simulink library "MyLib"  (R2024a)
settings: Solver=VariableStepAuto  StartTime=0.0  StopTime=10.0  RelTol=1e-3
values from neighbouring files (symbols this model uses):
  cnt_min = 10    [TX_PM_MODEL_Setup.m]
  cnt_n_bits = 9    [TX_PM_MODEL_Setup.m]
  R = 0.2    [TX_PM_MODEL_Setup.m]
  tcmp = 5    [TX_PM_MODEL_Setup.m]
undefined symbols (not defined in the file or in its folder): VDD_DRIVE
libraries: fl_lib x12, nesl_utility x7, $bdroot x3, ee_lib x1, spsTriangleGeneratorLib x1
settings Model: Creator=ciano  LastModifiedBy=ciano

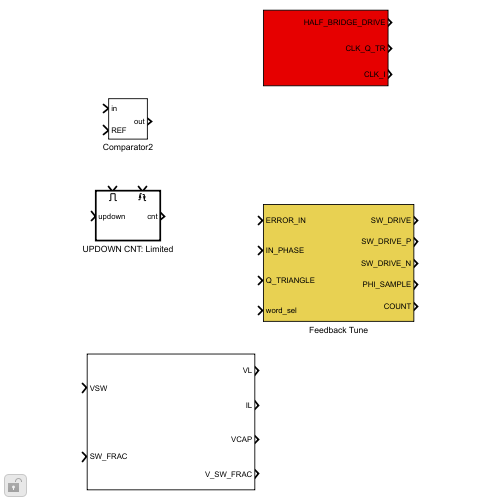
[thumbnail: Simulink's stored preview of the top-level diagram]
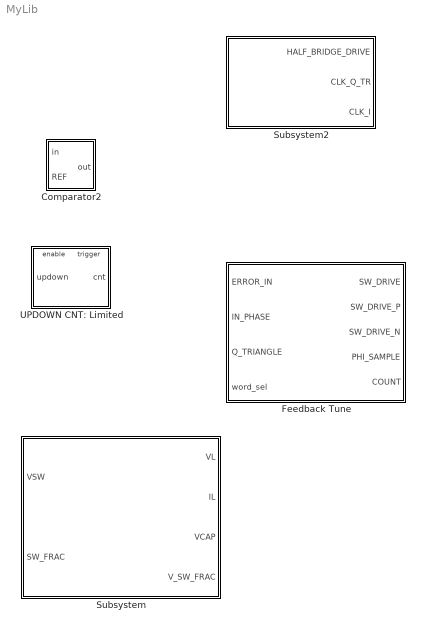
== system MyLib ==
  Comparator2 : Subsystem
  Feedback Tune : Subsystem
  Subsystem : Subsystem
  Subsystem2 : Subsystem
  UPDOWN CNT: Limited : Subsystem

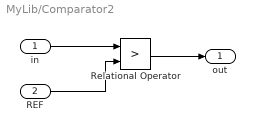
== system MyLib/Comparator2 ==
  in : Inport
  REF : Inport  Port=2
  Relational Operator : RelationalOperator  Operator=>  OutDataTypeStr=boolean  RndMeth=Simplest  InputSameDT=off
  out : Outport
  wires:
  in/1 -> Relational Operator/1
  Relational Operator/1 -> out/1
  REF/1 -> Relational Operator/2

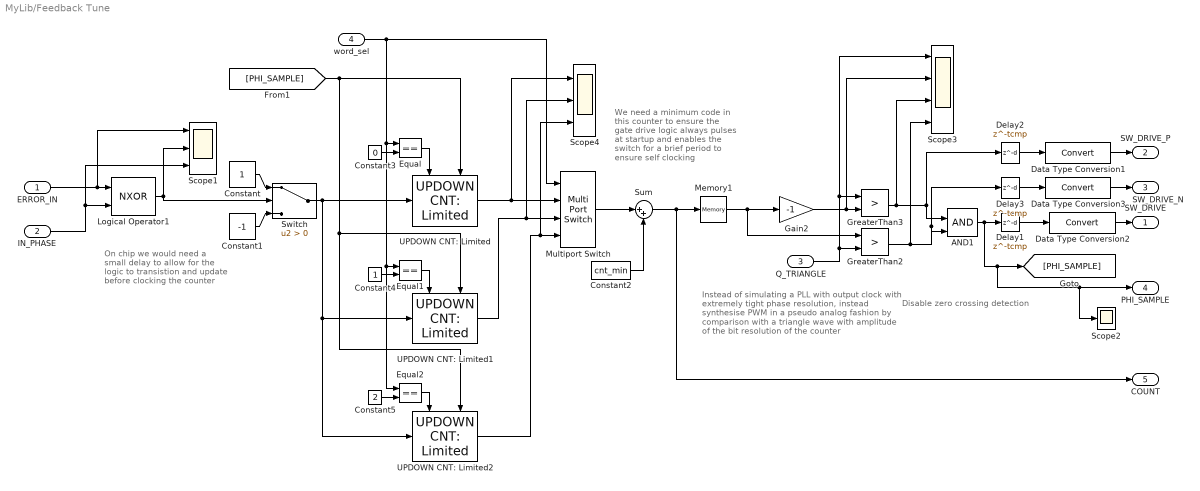
== system MyLib/Feedback Tune ==
  note: On chip we would need a small delay to allow for the logic to transistion and update before clocking the counter
  note: Instead of simulating a PLL with output clock with extremely tight phase resolution, instead synthesise PWM in a pseudo analog fashion by comparison with a triangle wave with amplitude of the bit resolution of the counter
  note: Disable zero crossing detection
  note: We need a minimum code in this counter to ensure the gate drive logic always pulses at startup and enables the switch for a brief period to ensure self clocking
  ERROR_IN : Inport
  IN_PHASE : Inport  Port=2
  Q_TRIANGLE : Inport  Port=3
  word_sel : Inport  Port=4
  AND1 : Logic  IconShape=distinctive  AllPortsSameDT=off  OutDataTypeStr=boolean
  Constant : Constant
  Constant1 : Constant  Value=-1
  Constant2 : Constant  Value=cnt_min
  Constant3 : Constant  Value=0
  Constant4 : Constant
  Constant5 : Constant  Value=2
  Data Type Conversion1 : DataTypeConversion  SaturateOnIntegerOverflow=off  RndMeth=Floor
  Data Type Conversion2 : DataTypeConversion  SaturateOnIntegerOverflow=off  RndMeth=Floor
  Data Type Conversion3 : DataTypeConversion  SaturateOnIntegerOverflow=off  RndMeth=Floor
  Delay1 : Delay  DelayLength=tcmp  SampleTime=1e-9
  Delay2 : Delay  DelayLength=tcmp  SampleTime=1e-9
  Delay3 : Delay  DelayLength=tcmp  SampleTime=1e-9
  Equal : RelationalOperator  Operator===  OutDataTypeStr=boolean  RndMeth=Simplest  InputSameDT=off
  Equal1 : RelationalOperator  Operator===  OutDataTypeStr=boolean  RndMeth=Simplest  InputSameDT=off
  Equal2 : RelationalOperator  Operator===  OutDataTypeStr=boolean  RndMeth=Simplest  InputSameDT=off
  Gain2 : Gain  Gain=-1
  GreaterThan2 : RelationalOperator  Operator=>  OutDataTypeStr=boolean  ZeroCross=off  RndMeth=Simplest  InputSameDT=off
  GreaterThan3 : RelationalOperator  Operator=>  OutDataTypeStr=boolean  ZeroCross=off  RndMeth=Simplest  InputSameDT=off
  Logical Operator1 : Logic  Operator=NXOR  IconShape=distinctive  AllPortsSameDT=off  OutDataTypeStr=boolean
  Memory1 : Memory
  Multiport Switch : MultiPortSwitch  DataPortOrder=Zero-based contiguous  zeroidx=on  SaturateOnIntegerOverflow=off  InputSameDT=off
  Scope1 : Scope  NumInputPorts=3
  Scope2 : Scope
  Scope3 : Scope  NumInputPorts=4
  Scope4 : Scope  NumInputPorts=3
  Sum : Sum  Inputs=|++
  Switch : Switch  Criteria=u2 > Threshold  ZeroCross=off  SaturateOnIntegerOverflow=off  InputSameDT=off
  UPDOWN CNT: Limited : $bdroot/UPDOWN CNT: Limited  SystemSampleTime=-1  VariantActivationTime=update diagram  AllowFlexibleInterface=on  Latency=0  AutoFrameSizeCalculation=off
  UPDOWN CNT: Limited1 : $bdroot/UPDOWN CNT: Limited  SystemSampleTime=-1  VariantActivationTime=update diagram  AllowFlexibleInterface=on  Latency=0  AutoFrameSizeCalculation=off
  UPDOWN CNT: Limited2 : $bdroot/UPDOWN CNT: Limited  SystemSampleTime=-1  VariantActivationTime=update diagram  AllowFlexibleInterface=on  Latency=0  AutoFrameSizeCalculation=off
  SW_DRIVE : Outport
  SW_DRIVE_P : Outport  Port=2
  SW_DRIVE_N : Outport  Port=3
  PHI_SAMPLE : Outport  Port=4
  COUNT : Outport  Port=5
  wires:
  Gain2/1 -> GreaterThan3/2, Scope3/2
  UPDOWN CNT: Limited/1 -> Scope4/1, Multiport Switch/2
  Switch/1 -> UPDOWN CNT: Limited/1, UPDOWN CNT: Limited2/1, UPDOWN CNT: Limited1/1
  Constant/1 -> Switch/1
  Constant1/1 -> Switch/3
  Logical Operator1/1 -> Switch/2, Scope1/2
  Data Type Conversion3/1 -> SW_DRIVE_N/1
  Data Type Conversion1/1 -> SW_DRIVE_P/1
  Delay3/1 -> Data Type Conversion3/1
  Delay2/1 -> Data Type Conversion1/1
  IN_PHASE/1 -> Logical Operator1/2, Scope1/3
  Data Type Conversion2/1 -> SW_DRIVE/1
  GreaterThan2/1 -> AND1/2, Delay3/1, Scope3/4
  AND1/1 -> Delay1/1, Scope2/1, PHI_SAMPLE/1, [PHI_SAMPLE]
  GreaterThan3/1 -> Delay2/1, AND1/1, Scope3/3
  Q_TRIANGLE/1 -> GreaterThan3/1, Scope3/1, GreaterThan2/2
  ERROR_IN/1 -> Logical Operator1/1, Scope1/1
  Delay1/1 -> Data Type Conversion2/1
  Memory1/1 -> Gain2/1, GreaterThan2/1
  word_sel/1 -> Equal2/1, Equal1/1, Equal/1, Multiport Switch/1
  Constant2/1 -> Sum/2
  Multiport Switch/1 -> Sum/1
  Sum/1 -> COUNT/1, Memory1/1
  [PHI_SAMPLE] -> UPDOWN CNT: Limited/Trigger, UPDOWN CNT: Limited2/Trigger, UPDOWN CNT: Limited1/Trigger
  UPDOWN CNT: Limited1/1 -> Scope4/2, Multiport Switch/3
  UPDOWN CNT: Limited2/1 -> Scope4/3, Multiport Switch/4
  Constant3/1 -> Equal/2
  Equal/1 -> UPDOWN CNT: Limited/Enable
  Constant4/1 -> Equal1/2
  Equal1/1 -> UPDOWN CNT: Limited1/Enable
  Equal2/1 -> UPDOWN CNT: Limited2/Enable
  Constant5/1 -> Equal2/2

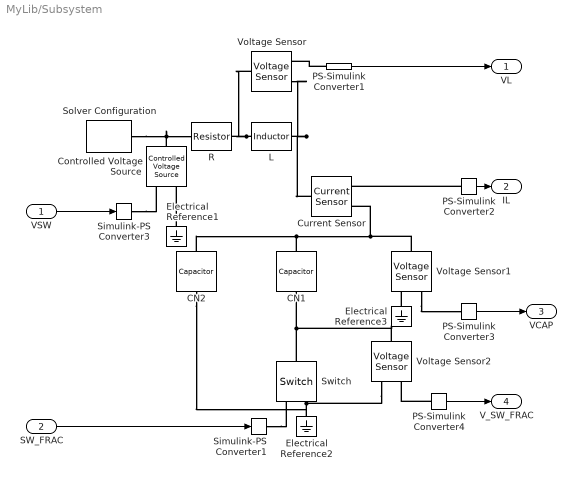
== system MyLib/Subsystem ==
  VSW : Inport
  SW_FRAC : Inport  Port=2
  CN1 : fl_lib/Electrical/Electrical Elements/Capacitor  c=3e-9 F  r=1e-6 Ohm  g=0 1/Ohm  i_specify=off  i_priority=None  i=0 A  i_nominal_specify=off  i_nominal_value=1  i_nominal_unit=A  v_specify=off  v_priority=None  v=0 V  v_nominal_specify=off  v_nominal_value=1  v_nominal_unit=V  vc_specify=off  vc_priority=High  vc=0 V  vc_nominal_specify=off  vc_nominal_value=1  vc_nominal_unit=V
  CN2 : fl_lib/Electrical/Electrical Elements/Capacitor  c=3e-9 F  r=1e-6 Ohm  g=0 1/Ohm  i_specify=off  i_priority=None  i=0 A  i_nominal_specify=off  i_nominal_value=1  i_nominal_unit=A  v_specify=off  v_priority=None  v=0 V  v_nominal_specify=off  v_nominal_value=1  v_nominal_unit=V  vc_specify=off  vc_priority=High  vc=0 V  vc_nominal_specify=off  vc_nominal_value=1  vc_nominal_unit=V
  Controlled Voltage Source : fl_lib/Electrical/Electrical Sources/Controlled Voltage Source
  Current Sensor : fl_lib/Electrical/Electrical Sensors/Current Sensor
  Electrical Reference1 : fl_lib/Electrical/Electrical Elements/Electrical Reference
  Electrical Reference2 : fl_lib/Electrical/Electrical Elements/Electrical Reference
  Electrical Reference3 : fl_lib/Electrical/Electrical Elements/Electrical Reference
  L : ee_lib/Passive/Inductor  l=L H  enable_L_tol=ee.enum.toleranceApplication.none  L_tol=20  tol_distribution=ee.enum.toleranceDistribution.uniform  nSigma=4  r=0 Ohm  g=1e-9 1/Ohm  enable_operating_limits=ee.enum.enable.no  operating_limit_action=ee.enum.passive.reportOpLim.warn  max_working_current=1 A  power_rating=1 W  enable_faults=ee.enum.enable.no  fault_action=simscape.enum.assert.action.none  lambdaPercent=50  k_faulted=0.9999  turnsShort=ee.enum.passive.inductor.turnsShortOption.no  openCct=ee.enum.enable.no  groundShort=ee.enum.passive.inductor.groundShortOption.no  groundShortG=0 1/Ohm  tau_fault=1e-3 s  fault_trigger=ee.enum.faults.faultTrigger.temporal  t_fault=1 s  max_permissible_voltage=100 V  n_fail_on_voltage=1  max_permissible_current=1 A  t_fail_on_current=1 s  i_L_specify=off  i_L_priority=High  i_L=0 A  i_L_nominal_specify=off  i_L_nominal_value=1  i_L_nominal_unit=A  faulted_specify=off  faulted_priority=None  faulted=0
  PS-Simulink Converter{1..4} (4 alike) : nesl_utility/PS-Simulink Converter  PhysicalDomain=network_engine_domain  SubClassName=ps_output  LeftPortType=input  RightPortType=output  PseudoPeriodic=off  Frequencies=[]  VectorFormat=inherit  Unit=inherit  AffineConversion=off
  R : fl_lib/Electrical/Electrical Elements/Resistor  R=R Ohm  i_specify=off  i_priority=None  i=0 A  i_nominal_specify=off  i_nominal_value=1  i_nominal_unit=A  v_specify=off  v_priority=None  v=0 V  v_nominal_specify=off  v_nominal_value=1  v_nominal_unit=V
  Simulink-PS Converter1 : nesl_utility/Simulink-PS Converter  PhysicalDomain=network_engine_domain  SubClassName=ps_input  LeftPortType=input  RightPortType=output  PseudoPeriodic=off  Frequencies=[]  NoiseDistribution=none  NoiseParameters=[]  Unit=1  AffineConversion=off  FilteringAndDerivatives=provide  SimscapeFilterOrder=1  InputFilterTimeConstant=0.001  UdotUserProvided=0
  Simulink-PS Converter3 : nesl_utility/Simulink-PS Converter  PhysicalDomain=network_engine_domain  SubClassName=ps_input  LeftPortType=input  RightPortType=output  PseudoPeriodic=off  Frequencies=[]  NoiseDistribution=none  NoiseParameters=[]  Unit=1  AffineConversion=off  FilteringAndDerivatives=provide  SimscapeFilterOrder=1  InputFilterTimeConstant=0.001  UdotUserProvided=0
  Solver Configuration : nesl_utility/Solver Configuration  PhysicalDomain=network_engine_domain  SubClassName=solver  LeftPortType=input  RightPortType=generic  Tones=[]  Harmonics=[]  SimulateNoise=off  Profile=off  UseLocalSampling=off  EnableSwitchedLinearOptims=on  FrequencyDomain=off  UseCCode=off  RelTol=0.001  AbsTol=0.001  MinStep=1e-09  ToWorkspace=off  RevertToSquareIcSolve=off  NumHomotopyIterations=100  PhasorMode=off  PhasorModeNumHarmonics=1  ConsistencySolver=NEWTON_XTOL_AFTER_FTOL  IndexReductionMethod=DerivativeReplacement  DoDC=off  ResidualTolerance=1e-09  ConsistencyTolSource=GLOBAL  ConsistencyAbsTol=0.001  ConsistencyRelTol=0.001  ConsistencyTolFactor=0.001  UseLocalSolver=off  LocalSolverChoice=NE_BACKWARD_EULER_ADVANCER  ResolveIndetEquations=on  FunctionEvalNumThread=1  LocalSolverSampleTime=0.001  DoFixedCost=off  MaxNonlinIter=3  MaxModeIter=2  ComputeImpulses=off  ImpulseIterations=2  LinearAlgebra=auto  LinearAlgebraNumThread=0  EquationFormulation=NE_TIME_EF  DelaysMemoryBudget=1024  AutomaticFiltering=on  FilteringTimeConstant=0.001  PartitionStorageMethod=AS_NEEDED  PartitionMemoryBudget=1024  PartitionMethod=ROBUST  MultibodyUseLocalSolver=off  MultibodyLocalSolverChoice=ODE1  MultibodyLocalSolverSampleTime=0.001
  Switch : fl_lib/Electrical/Electrical Elements/Switch  R_closed=0.01 Ohm  G_open=1e-8 1/Ohm  Threshold=0.5  i_specify=off  i_priority=None  i=0 A  i_nominal_specify=off  i_nominal_value=1  i_nominal_unit=A  v_specify=off  v_priority=None  v=0 V  v_nominal_specify=off  v_nominal_value=1  v_nominal_unit=V
  Voltage Sensor : fl_lib/Electrical/Electrical Sensors/Voltage Sensor
  Voltage Sensor1 : fl_lib/Electrical/Electrical Sensors/Voltage Sensor
  Voltage Sensor2 : fl_lib/Electrical/Electrical Sensors/Voltage Sensor
  VL : Outport
  IL : Outport  Port=2
  VCAP : Outport  Port=3
  V_SW_FRAC : Outport  Port=4
  wires:
  PS-Simulink Converter1/1 -> VL/1
  VSW/1 -> Simulink-PS Converter3/1
  PS-Simulink Converter4/1 -> V_SW_FRAC/1
  PS-Simulink Converter2/1 -> IL/1
  SW_FRAC/1 -> Simulink-PS Converter1/1
  PS-Simulink Converter3/1 -> VCAP/1
  connections:
  Solver Configuration/RConn1 -- R/LConn1 -- Controlled Voltage Source/LConn1
  R/RConn1 -- Voltage Sensor/LConn1 -- L/LConn1
  PS-Simulink Converter4/LConn1 -- Voltage Sensor2/RConn1
  Simulink-PS Converter1/RConn1 -- Switch/RConn1
  Voltage Sensor2/RConn2 -- Switch/RConn2 -- CN2/RConn1 -- Electrical Reference2/LConn1
  PS-Simulink Converter1/LConn1 -- Voltage Sensor/RConn1
  PS-Simulink Converter2/LConn1 -- Current Sensor/RConn1
  CN2/LConn1 -- Current Sensor/RConn2 -- Voltage Sensor1/LConn1 -- CN1/LConn1
  Simulink-PS Converter3/RConn1 -- Controlled Voltage Source/RConn1
  Switch/LConn1 -- Voltage Sensor2/LConn1 -- CN1/RConn1
  Electrical Reference3/LConn1 -- Voltage Sensor1/RConn2
  Voltage Sensor1/RConn1 -- PS-Simulink Converter3/LConn1
  Electrical Reference1/LConn1 -- Controlled Voltage Source/RConn2
  L/RConn1 -- Voltage Sensor/RConn2 -- Current Sensor/LConn1

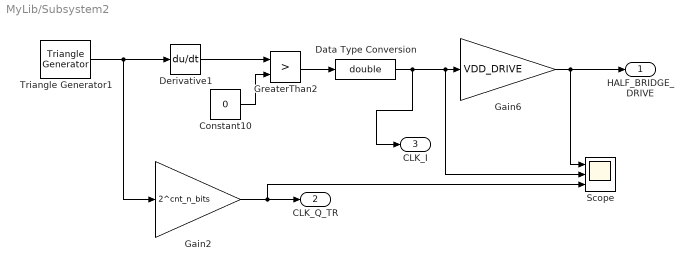
== system MyLib/Subsystem2 ==
  Constant10 : Constant  Value=0
  Data Type Conversion : DataTypeConversion  OutDataTypeStr=double  SaturateOnIntegerOverflow=off  RndMeth=Floor
  Derivative1 : Derivative
  Gain2 : Gain  Gain=2^cnt_n_bits
  Gain6 : Gain  Gain=VDD_DRIVE
  GreaterThan2 : RelationalOperator  Operator=>  OutDataTypeStr=boolean  RndMeth=Simplest  InputSameDT=off
  Scope : Scope  NumInputPorts=3
  Triangle Generator1 : spsTriangleGeneratorLib/Triangle Generator  Freq=fin  Phase=90  Ts=0
  HALF_BRIDGE_DRIVE : Outport
  CLK_Q_TR : Outport  Port=2
  CLK_I : Outport  Port=3
  wires:
  Data Type Conversion/1 -> Gain6/1, Scope/2, CLK_I/1
  Constant10/1 -> GreaterThan2/2
  GreaterThan2/1 -> Data Type Conversion/1
  Derivative1/1 -> GreaterThan2/1
  Gain2/1 -> CLK_Q_TR/1, Scope/3
  Gain6/1 -> HALF_BRIDGE_DRIVE/1, Scope/1
  Triangle Generator1/1 -> Gain2/1, Derivative1/1

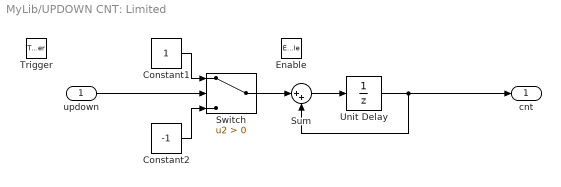
== system MyLib/UPDOWN CNT: Limited ==
  updown : Inport
  Enable : EnablePort
  Trigger : TriggerPort  TriggerType=either  VariantControl=(inherit)  PortDimensions=1
  Constant1 : Constant
  Constant2 : Constant  Value=-1
  Sum : Sum  Inputs=|++
  Switch : Switch  Criteria=u2 > Threshold  SaturateOnIntegerOverflow=off  InputSameDT=off
  Unit Delay : UnitDelay  SampleTime=-1  HasFrameUpgradeWarning=on
  cnt : Outport
  wires:
  Unit Delay/1 -> Sum/2, cnt/1
  Constant1/1 -> Switch/1
  updown/1 -> Switch/2
  Sum/1 -> Unit Delay/1
  Constant2/1 -> Switch/3
  Switch/1 -> Sum/1
